simulink model "MFSK"  (R2016b)
settings: Solver=FixedStepDiscrete  StartTime=0.0  StopTime=1000*(1/10E3)  FixedStep=1/10E3  RelTol=1e-3
values from neighbouring files (symbols this model uses):
  M = 2    [var.m]
  N = 2    [var.m]
libraries: commdigbbndfm2 x3, commdigbbndpm3 x2, commdigbbndam3 x2, commchan3 x1, commrandsrc3 x1, commsink2 x1
settings Model: Creator=ak22070  LastModifiedBy=ak22070
settings DataIOCC: ExternalInput=[N]  SaveOutput=off  OutputSaveName=Ber

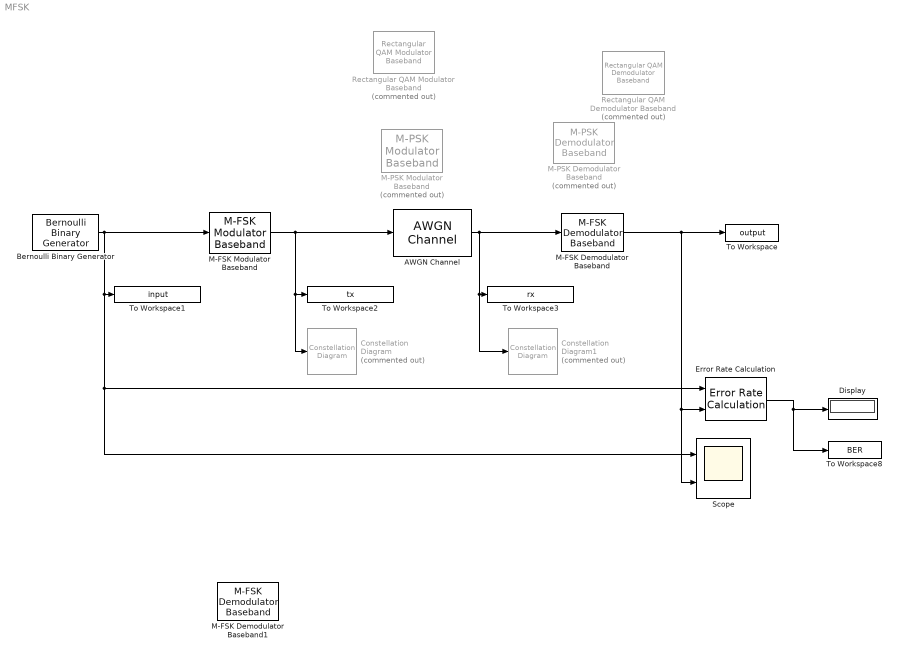
== system MFSK ==
  AWGN Channel : commchan3/AWGN Channel  InputProcessing=Columns as channels (frame based)  seed=67  noiseMode="Signal to noise ratio  (Eb/No)"  EbNodB=EbNo  EsNodB=EbNo  SNRdB=10  bitsPerSym=N  Ps=1  Tsym=N  variance=1
  Bernoulli Binary Generator : commrandsrc3/Bernoulli Binary Generator  ProbabilityOfZero=0.5  SeedSource=Auto  Seed=0  SampleTime=1  SamplesPerFrame=N*1000  OutputDataType=double  SimulateUsing=Interpreted execution
  Constellation Diagram : ConstellationDiagram  Commented=on
  Constellation Diagram1 : ConstellationDiagram  Commented=on
  Display : Display
  Error Rate Calculation : commsink2/Error Rate Calculation  N=0  st_delay=0  cp_mode=Entire frame  subframe=[]  PMode=Port  WsName=Ber  RsMode2=off  stop=on  numErr=maxNumErrs  maxBits=maxNumBits
  M-FSK Demodulator Baseband : commdigbbndfm2/M-FSK Demodulator Baseband  M=M  OutType=Bit  Dec=Gray  freqSep=F_sep  numSamp=N  RateOptions=Enforce single-rate processing  outDataType=double
  M-FSK Demodulator Baseband1 : commdigbbndfm2/M-FSK Demodulator Baseband  M=8  OutType=Integer  Dec=Gray  freqSep=6  numSamp=17  RateOptions=Enforce single-rate processing  outDataType=double
  M-FSK Modulator Baseband : commdigbbndfm2/M-FSK Modulator Baseband  M=M  InType=Bit  Enc=Gray  freqSep=F_sep  phaseType=Continuous  numSamp=N  RateOptions=Enforce single-rate processing  outDataType=double
  M-PSK Demodulator Baseband : commdigbbndpm3/M-PSK Demodulator Baseband  Commented=on  M=M  OutType=Bit  DecType=Hard decision  VarSource=Dialog  Variance=1  Dec=Gray  Mapping=[0:7]  Ph=pi/M  outDtype1=Inherit via internal rule  outDtype2=double  derotateFactorWordLen=16  derotateFactorDataTypeStr=Inherit: Same word length as input  derotateFactorLastDataTypeStr=Inherit: Same word length as input
  M-PSK Modulator Baseband : commdigbbndpm3/M-PSK Modulator Baseband  Commented=on  M=M  InType=Bit  Enc=Gray  Mapping=[0:7]  Ph=pi/M  outDtype=double  outWordLen=16  outUDDataType=sfix(16)  outFracLenMode=Best precision  outFracLen=15  outDataTypeStr=double  outLastDataTypeStr=double
  Rectangular QAM Demodulator Baseband : commdigbbndam3/Rectangular QAM Demodulator Baseband  Commented=on  M=M  OutType=Bit  DecType=Hard decision  VarSource=Dialog  Variance=1  Dec=Gray  Mapping=[0:15]  PowType=Min. distance between symbols  MinDist=dmin  AvgPow=1  PeakPow=1  Ph=0  outDtype1=Inherit via internal rule  outDtype2=Inherit via internal rule  derotateFactorWordLen=16  derotateFactorDataTypeStr=Inherit: Same word length as input  derotateFactorLastDataTypeStr=Inherit: Same word length as input  denormFactorWordLen=16  denormFactorDataTypeStr=Inherit: Same word length as input  denormFactorLastDataTypeStr=Inherit: Same word length as input  prodOutWordLen=32  prodOutOverflowMode=Wrap  prodOutRoundingMode=Floor  prodOutOvFlMode=off  prodOutOvFlModeLastStrValue=off  sumWordLen=32
  Rectangular QAM Modulator Baseband : commdigbbndam3/Rectangular QAM Modulator Baseband  Commented=on  M=M  InType=Bit  Enc=Gray  Mapping=[0:15]  PowType=Min. distance between symbols  MinDist=dmin  AvgPow=1  PeakPow=1  Ph=0  outDtype=double  outWordLen=16  outUDDataType=sfix(16)  outFracLenMode=Best precision  outFracLen=15  outDataTypeStr=double  outLastDataTypeStr=double
  Scope : Scope  NumInputPorts=2
  To Workspace : ToWorkspace  VariableName=output  SaveFormat=Timeseries  SampleTime=-1
  To Workspace1 : ToWorkspace  VariableName=input  SaveFormat=Timeseries  SampleTime=-1
  To Workspace2 : ToWorkspace  VariableName=tx  SaveFormat=Timeseries  SampleTime=-1
  To Workspace3 : ToWorkspace  VariableName=rx  SaveFormat=Timeseries  SampleTime=-1
  To Workspace8 : ToWorkspace  VariableName=BER  SampleTime=-1
      settings: MaxDataPoints=1  Save2DSignal=2-D array (concatenate along first dimension)
  wires:
  Bernoulli Binary Generator/1 -> M-FSK Modulator Baseband/1, To Workspace1/1, Scope/1, Error Rate Calculation/1
  M-FSK Demodulator Baseband/1 -> Scope/2, Error Rate Calculation/2, To Workspace/1
  AWGN Channel/1 -> M-FSK Demodulator Baseband/1, Constellation Diagram1/1, To Workspace3/1
  Error Rate Calculation/1 -> Display/1, To Workspace8/1
  M-FSK Modulator Baseband/1 -> Constellation Diagram/1, To Workspace2/1, AWGN Channel/1
